simulink model "wheel_loader_simscape"  (R2026a)
settings: configuration reference "standardSILConfiguraitonParams" (kept outside this file)
libraries: nesl_utility x3, fl_lib x3, ee_lib x1
settings Model: Creator=jerem  LastModifiedBy=Usuario
settings ConfigSetRef: SourceName=standardSILConfiguraitonParams  SourceLocation=Base Workspace

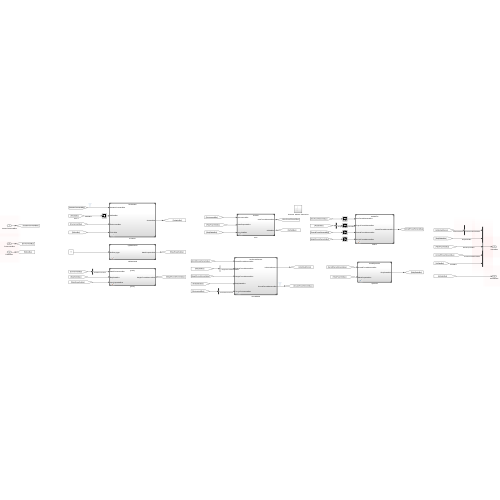
[thumbnail: Simulink's stored preview of the top-level diagram]
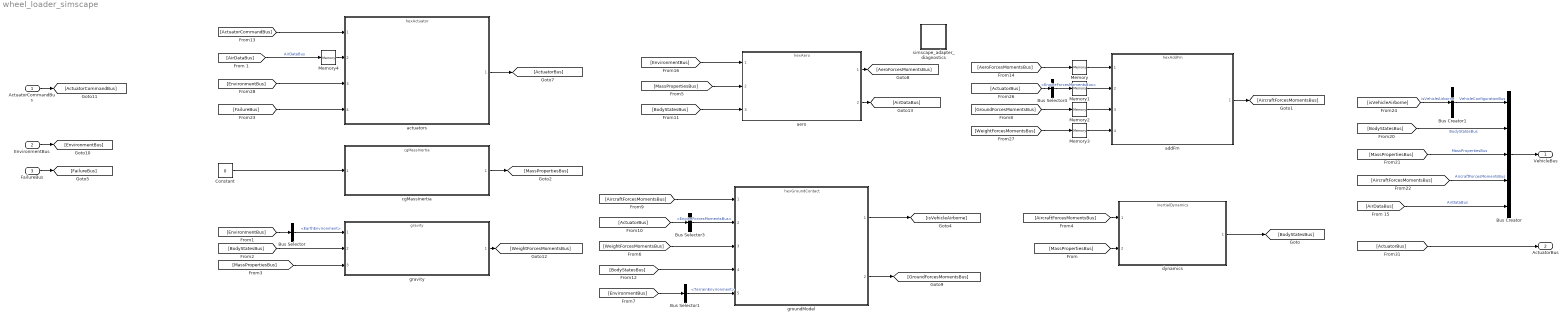
== system wheel_loader_simscape ==
  ActuatorCommandBus : Inport  OutDataTypeStr=Bus: ActuatorCommandBus
  EnvironmentBus : Inport  Port=2  OutDataTypeStr=Bus: EnvironmentBus
  FailureBus : Inport  Port=3  OutDataTypeStr=Bus: FailureBus
  Bus Creator : BusCreator  Inputs=5  OutDataTypeStr=Bus: VehicleBus
  Bus Creator1 : BusCreator  Inputs=1  OutDataTypeStr=Bus: VehicleConfigurationBus
  Bus Selector : BusSelector  OutputSignals=EarthEnvironment
  Bus Selector1 : BusSelector  OutputSignals=TerrainEnvironment
  Bus Selector3 : BusSelector  OutputSignals=PropulsionBus.EngineForcesMomentsBus
  Bus Selector4 : BusSelector  OutputSignals=PropulsionBus.EngineForcesMomentsBus
  Constant : Constant  Value=0
  Memory{,1..4} (5 alike) : Memory
  actuators : ModelReference  ModelNameDialog=hexActuator.slx  SimulationMode=Normal  ModelReferenceVersion=1.37
  addFm : ModelReference  ModelNameDialog=hexAddFm.slx  SimulationMode=Normal  ModelReferenceVersion=1.14
  aero : ModelReference  ModelNameDialog=hexAero.slx  SimulationMode=Normal  ModelReferenceVersion=1.17
  cgMassInertia : ModelReference  ModelNameDialog=cgMassInertia.slx  SimulationMode=Normal  ModelReferenceVersion=1.43
  dynamics : ModelReference  ModelNameDialog=inertialDynamics.slx  SimulationMode=Normal  ModelReferenceVersion=1.35
  gravity : ModelReference  ModelNameDialog=gravity.slx  SimulationMode=Normal  ModelReferenceVersion=1.28
  groundModel : ModelReference  ModelNameDialog=hexGroundContact.slx  SimulationMode=Normal  ModelReferenceVersion=5.2
  simscape_adapter_diagnostics : Subsystem
  VehicleBus : Outport  OutDataTypeStr=Bus: VehicleBus
  ActuatorBus : Outport  Port=2  OutDataTypeStr=Bus: ActuatorBus
  wires:
  Bus Creator1/1 -> Bus Creator/1  "VehicleConfigurationBus"
  [isVehicleAirborne] -> Bus Creator1/1  "isVehicleAirborne"
  [MassPropertiesBus] -> Bus Creator/3  "MassPropertiesBus"
  [AircraftForcesMomentsBus] -> Bus Creator/4  "AircraftForcesMomentsBus"
  [BodyStatesBus] -> Bus Creator/2  "BodyStatesBus"
  Bus Creator/1 -> VehicleBus/1
  [AirDataBus] -> Bus Creator/5  "AirDataBus"
  dynamics/1 -> [BodyStatesBus]
  [AircraftForcesMomentsBus] -> dynamics/1
  addFm/1 -> [AircraftForcesMomentsBus]
  cgMassInertia/1 -> [MassPropertiesBus]
  [MassPropertiesBus] -> dynamics/2
  ActuatorCommandBus/1 -> [ActuatorCommandBus]
  EnvironmentBus/1 -> [EnvironmentBus]
  [EnvironmentBus] -> Bus Selector/1
  Bus Selector/1 -> gravity/1  "<EarthEnvironment>"
  [BodyStatesBus] -> gravity/2
  [MassPropertiesBus] -> gravity/3
  gravity/1 -> [WeightForcesMomentsBus]
  Constant/1 -> cgMassInertia/1
  Memory4/1 -> actuators/2
  [EnvironmentBus] -> actuators/3
  [ActuatorCommandBus] -> actuators/1
  [AirDataBus] -> Memory4/1  "AirDataBus"
  actuators/1 -> [ActuatorBus]
  [BodyStatesBus] -> aero/3
  [MassPropertiesBus] -> aero/2
  [EnvironmentBus] -> aero/1
  [AeroForcesMomentsBus] -> Memory/1
  [ActuatorBus] -> Bus Selector4/1
  [GroundForcesMomentsBus] -> Memory2/1
  [WeightForcesMomentsBus] -> Memory3/1
  groundModel/1 -> [isVehicleAirborne]
  groundModel/2 -> [GroundForcesMomentsBus]
  Bus Selector1/1 -> groundModel/5  "<TerrainEnvironment>"
  [WeightForcesMomentsBus] -> groundModel/3
  aero/2 -> [AirDataBus]
  aero/1 -> [AeroForcesMomentsBus]
  Bus Selector4/1 -> Memory1/1  "<EngineForcesMomentsBus>"
  FailureBus/1 -> [FailureBus]
  [FailureBus] -> actuators/4
  [ActuatorBus] -> ActuatorBus/1
  [EnvironmentBus] -> Bus Selector1/1
  Bus Selector3/1 -> groundModel/2  "<EngineForcesMomentsBus>"
  [ActuatorBus] -> Bus Selector3/1
  [BodyStatesBus] -> groundModel/4
  [AircraftForcesMomentsBus] -> groundModel/1
  Memory1/1 -> addFm/2
  Memory2/1 -> addFm/3
  Memory3/1 -> addFm/4
  Memory/1 -> addFm/1

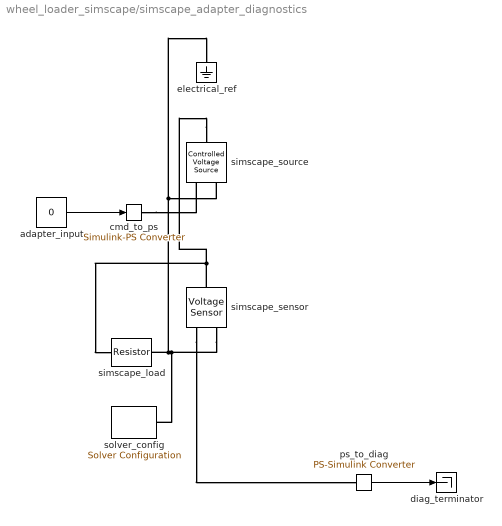
== system wheel_loader_simscape/simscape_adapter_diagnostics ==
  adapter_input : Constant  Value=0
  cmd_to_ps : nesl_utility/Simulink-PS Converter  PhysicalDomain=network_engine_domain  SubClassName=ps_input  LeftPortType=input  RightPortType=output  PseudoPeriodic=off  Frequencies=[]  NoiseDistribution=none  NoiseParameters=[]  Unit=1  AffineConversion=off  FilteringAndDerivatives=provide  SimscapeFilterOrder=1  InputFilterTimeConstant=0.001  UdotUserProvided=0
  diag_terminator : Terminator
  electrical_ref : fl_lib/Electrical/Electrical Elements/Electrical Reference
  ps_to_diag : nesl_utility/PS-Simulink Converter  PhysicalDomain=network_engine_domain  SubClassName=ps_output  LeftPortType=input  RightPortType=output  PseudoPeriodic=off  Frequencies=[]  VectorFormat=inherit  Unit=inherit  AffineConversion=off
  simscape_load : ee_lib/Passive/Resistor  R=1 Ohm  enable_R_tol=ee.enum.toleranceApplication.none  R_tol=5  tol_distribution=ee.enum.toleranceDistribution.uniform  nSigma=4  enable_operating_limits=ee.enum.enable.no  operating_limit_action=ee.enum.passive.reportOpLim.warn  power_rating=1 W  max_working_voltage=100 V  noise_mode=ee.enum.sources.noise.Disabled  Tdevice=25 degC  sample_time=1e-3 s  repeatability=ee.enum.ic.repeatability.notRepeatable  user_seed=0  auto_seed=545404223  power_derating_T1=70 degC  power_derating_T2=155 degC  operating_temperature_range_vec=[-50, 150] degC  alpha=3.93e-3 1/K  Tmeas=25 degC  thermal_mass=100 J/K  temperature_specify=off  temperature_priority=High  temperature=298.15 K  temperature_nominal_specify=off  temperature_nominal_value=1  temperature_nominal_unit=K
  simscape_sensor : fl_lib/Electrical/Electrical Sensors/Voltage Sensor
  simscape_source : fl_lib/Electrical/Electrical Sources/Controlled Voltage Source
  solver_config : nesl_utility/Solver Configuration  PhysicalDomain=network_engine_domain  SubClassName=solver  LeftPortType=input  RightPortType=generic  Tones=[]  Harmonics=[]  SimulateNoise=off  Profile=off  UseLocalSampling=off  EnableSwitchedLinearOptims=on  FrequencyDomain=off  UseCCode=off  RelTol=0.001  AbsTol=0.001  MinStep=1e-09  ToWorkspace=off  RevertToSquareIcSolve=off  NumHomotopyIterations=100  PhasorMode=off  PhasorModeNumHarmonics=1  ConsistencySolver=NEWTON_XTOL_AFTER_FTOL  CanonicalOrdering=CANONICAL  OptimizeIntermediates=OPTIMIZED  IndexReductionMethod=DerivativeReplacement  DoDC=off  ResidualTolerance=1e-09  ConsistencyTolSource=GLOBAL  ConsistencyAbsTol=0.001  ConsistencyRelTol=0.001  ConsistencyTolFactor=0.001  UseLocalSolver=off  LocalSolverChoice=NE_BACKWARD_EULER_ADVANCER  ResolveIndetEquations=on  FunctionEvalNumThread=1  LocalSolverSampleTime=0.001  DoFixedCost=off  MaxNonlinIter=3  MaxModeIter=2  ComputeImpulses=off  ImpulseIterations=2  LinearAlgebra=auto  LinearAlgebraNumThread=0  EquationFormulation=NE_TIME_EF  DelaysMemoryBudget=1024  AutomaticFiltering=on  FilteringTimeConstant=0.001  PartitionStorageMethod=AS_NEEDED  PartitionMemoryBudget=1024  PartitionMethod=ROBUST  MultibodyUseLocalSolver=off  MultibodyLocalSolverChoice=ODE1  MultibodyLocalSolverSampleTime=0.001
  wires:
  ps_to_diag/1 -> diag_terminator/1
  adapter_input/1 -> cmd_to_ps/1
  connections:
  simscape_sensor/RConn1 -- ps_to_diag/LConn1
  simscape_source/RConn2 -- simscape_sensor/RConn2 -- solver_config/RConn1 -- simscape_load/RConn1 -- electrical_ref/LConn1
  simscape_source/LConn1 -- simscape_sensor/LConn1 -- simscape_load/LConn1
  cmd_to_ps/RConn1 -- simscape_source/RConn1
